simulink model "Realimentacion_Perturbacion2015"  (Simulink 8.6)
settings: Solver=VariableStepAuto  SolverMode=SingleTasking  StartTime=0.0  StopTime=30  RelTol=1e-3
values from neighbouring files (symbols this model uses):
  a = [0 1 0 0 ... (first row only)    [rejection_Disturbance.m]
  b = [0;1;0;-2]    [rejection_Disturbance.m]
  c = [1 0 0 0]    [rejection_Disturbance.m]
  k1 = K(1:end-1)    [rejection_Disturbance.m]
  k2 = -K(end)    [rejection_Disturbance.m]
settings Model: Creator=Sergio  LastModifiedBy=Sergio
settings DataIOCC: LimitDataPoints=off  SaveFormat=Dataset  SignalLoggingSaveFormat=Dataset  ReturnWorkspaceOutputs=on
settings OptimizationCC: ExpressionDepthLimit=128
settings DebuggingCC: UnderspecifiedInitializationDetection=Simplified  MergeDetectMultiDrivingBlocksExec=error  SolverPrmCheckMsg=none  FcnCallInpInsideContextMsg=EnableAllAsError  AllowSymbolicDim=on  StateNameClashWarn=none  SFUnexpectedBacktrackingDiag=error  SFNoUnconditionalDefaultTransitionDiag=error
settings HardwareCC: ProdBitPerPointer=64  ProdLargestAtomicFloat=Float  ProdIntDivRoundTo=Zero  ProdEndianess=LittleEndian  ProdWordSize=64  ProdHWDeviceType=Intel->x86-64 (Windows64)
settings ModelReferenceCC: PropagateSignalLabelsOutOfModel=on
settings SFSimCC: SimUseLocalCustomCode=on
settings RTWCC: RTWUseLocalCustomCode=on
settings GRTTargetCC: TargetLangStandard=C99 (ISO)  CombineOutputUpdateFcns=on  GRTInterface=off
settings ConfigComp: CovMetricSettings=dwe  CovHtmlReporting=off  CovSaveCumulativeToWorkspaceVar=off  CovSaveSingleToWorkspaceVar=off  CovExternalEMLEnable=on

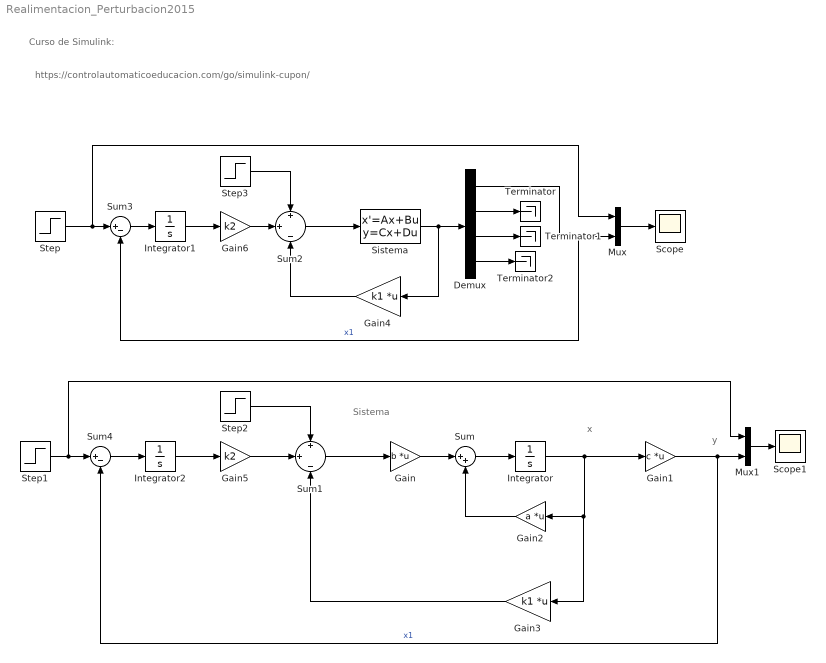
== system Realimentacion_Perturbacion2015 ==
  note: https://controlautomaticoeducacion.com/go/simulink-cupon/
  note: Curso de Simulink:
  note: y
  note: x
  note: Sistema
  Demux : Demux
  Gain : Gain  Gain=b  Multiplication=Matrix(K*u)
  Gain1 : Gain  Gain=c  Multiplication=Matrix(K*u)
  Gain2 : Gain  Gain=a  Multiplication=Matrix(K*u)
  Gain3 : Gain  Gain=k1  Multiplication=Matrix(K*u)
  Gain4 : Gain  Gain=k1  Multiplication=Matrix(K*u)
  Gain5 : Gain  Gain=k2
  Gain6 : Gain  Gain=k2
  Integrator : Integrator
  Integrator1 : Integrator
  Integrator2 : Integrator
  Mux : Mux  Inputs=2
  Mux1 : Mux  Inputs=2
  Scope : Scope
  Scope1 : Scope
  Sistema : StateSpace  A=a  B=b  C=eye(4)  D=[0;0;0;0]  X0=0
  Step : Step  SampleTime=0
  Step1 : Step  SampleTime=0
  Step2 : Step  Time=15  After=1.5  SampleTime=0
  Step3 : Step  Time=15  After=1.5  SampleTime=0
  Sum : Sum  Inputs=|++
  Sum1 : Sum  Inputs=+|+|-
  Sum2 : Sum  Inputs=+|+|-
  Sum3 : Sum  Inputs=|+-
  Sum4 : Sum  Inputs=|+-
  Terminator : Terminator
  Terminator1 : Terminator
  Terminator2 : Terminator
  wires:
  Gain/1 -> Sum/1
  Sum/1 -> Integrator/1
  Integrator/1 -> Gain3/1, Gain2/1, Gain1/1
  Gain2/1 -> Sum/2
  Step1/1 -> Sum4/1, Mux1/1
  Sum1/1 -> Gain/1
  Gain3/1 -> Sum1/3
  Sistema/1 -> Gain4/1, Demux/1
  Demux/2 -> Terminator/1
  Demux/3 -> Terminator1/1
  Demux/4 -> Terminator2/1
  Sum2/1 -> Sistema/1
  Gain4/1 -> Sum2/3
  Mux/1 -> Scope/1
  Step/1 -> Sum3/1, Mux/1
  Demux/1 -> Mux/2, Sum3/2  "x1"
  Gain1/1 -> Sum4/2, Mux1/2  "x1"
  Mux1/1 -> Scope1/1
  Sum4/1 -> Integrator2/1
  Integrator2/1 -> Gain5/1
  Gain6/1 -> Sum2/2
  Integrator1/1 -> Gain6/1
  Sum3/1 -> Integrator1/1
  Gain5/1 -> Sum1/2
  Step2/1 -> Sum1/1
  Step3/1 -> Sum2/1
